simulink model "frequence_response_1"  (R2021b)
settings: Solver=VariableStepAuto  StartTime=0.0  StopTime=30  RelTol=1e-3
values from neighbouring files (symbols this model uses):
  f1 = [2 2]    [main.m]    (also in main1.m)
  phi1 = [0 0]    [main.m]    (also in main1.m)
  U1_max = [3 6]    [main.m]    (also in main1.m)
undefined symbols (not defined in the file or in its folder): A, B, C, D
settings Model: Creator=PaoloA  LastModifiedBy=PaoloA

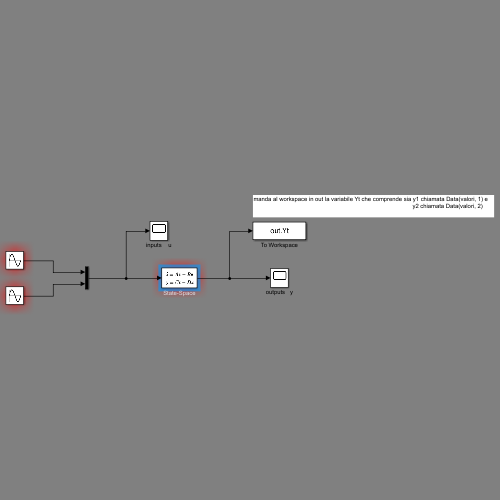
[thumbnail: Simulink's stored preview of the top-level diagram]
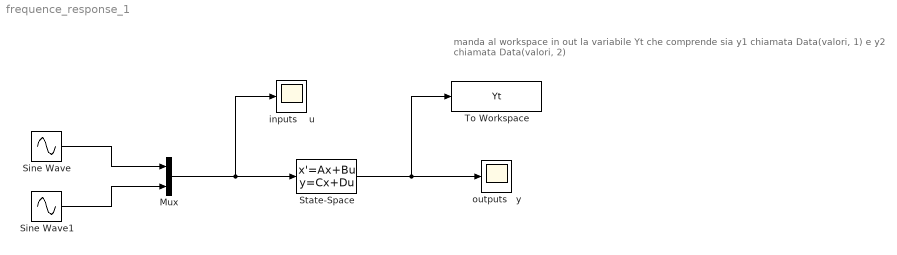
== system frequence_response_1 ==
  note: manda al workspace in out la variabile Yt che comprende sia y1 chiamata Data(valori, 1) e
      | 												           y2 chiamata Data(valori, 2)
  Mux : Mux  Inputs=2
  Sine Wave : Sin  Amplitude=U1_max(1)  Frequency=f1(1)  Phase=phi1(1)  SampleTime=0
  Sine Wave1 : Sin  Amplitude=U1_max(2)  Frequency=f1(2)  Phase=phi1(2)  SampleTime=0
  State-Space : StateSpace  A=A  B=B  C=C  D=D  InitialCondition=0
  To Workspace : ToWorkspace  VariableName=Yt  SaveFormat=Timeseries  SampleTime=-1
  inputs    u : Scope
  outputs   y : Scope
  wires:
  State-Space/1 -> To Workspace/1, outputs   y/1
  Mux/1 -> inputs    u/1, State-Space/1
  Sine Wave/1 -> Mux/1
  Sine Wave1/1 -> Mux/2
